simulink model "Target_Control_System"  (R2021b)
settings: Solver=FixedStepDiscrete  StartTime=0.0  StopTime=5  RelTol=1e-3
PreLoadFcn:
  | RTWConfigurationCB('preloadfcn', bdroot);
PostLoadFcn:
  | load('configuration/data_struct.mat');
  | load('configuration/fluxMaps_propMotor.mat');
  | load('configuration/parameterInit_PROP.mat');
  | load('configuration/parameterInit_PUMP.mat');
  | load('configuration/parameterInit_PITCH.mat');
  | load('configuration/parameterInit_TILT.mat');
  | %load('configuration/base_workspace_signal_definition.mat');
  | %load('resolvedatastores_to_baseworkspace_for_faster_simulation.mat');
model workspace (MAT data in the model file):
  SIMULATION_OPTIONS : Simulink.Parameter (value not decoded)
  TARGET_CODE_GEN : Simulink.Parameter (value not decoded)
  TCS_SAMPLE_FREQ_HZ : Simulink.Parameter (value not decoded)
symbols that are objects in the model workspace (value not decoded): TARGET_CODE_GEN, TCS_SAMPLE_FREQ_HZ
undefined symbols (not defined in the file): A_DQ_REF_LPF_INIT__PITCH, A_DQ_REF_LPF_INIT__PROP, A_DQ_REF_LPF_INIT__PUMP, A_DQ_REF_LPF_INIT__TILT, A_OBSERVER_CONFIDENCE_INIT__PITCH, A_OBSERVER_CONFIDENCE_INIT__PROP, A_OBSERVER_CONFIDENCE_INIT__PUMP, A_OBSERVER_CONFIDENCE_INIT__TILT, ACTUATOR_MAX_ANGLE_TRIP__PITCH, ACTUATOR_MIN_ANGLE_TRIP__PITCH, ACTUATOR_POS_SENSOR_INV_DIRECTION__PITCH, ACTUATOR_POS_SENSOR_INV_DIRECTION__TILT, ACTUATOR_POS_SENSOR_OFFSET__PITCH, ACTUATOR_POS_SENSOR_OFFSET__TILT, ADC_scaler1_baseaddr_TILT, ADC_SCALER_FLOAT_TO_FIXPOINT_EXPANSION, ANGLE_ELEC_FROM_SENSOR_OFFSET_INIT__PITCH, ANGLE_ELEC_FROM_SENSOR_OFFSET_INIT__PROP, ANGLE_ELEC_FROM_SENSOR_OFFSET_INIT__PUMP, ANGLE_ELEC_FROM_SENSOR_OFFSET_INIT__TILT, AUTO_CLEAR_FAULTS_ENABLED__PITCH, AUTO_CLEAR_FAULTS_ENABLED__PROP, AUTO_CLEAR_FAULTS_ENABLED__PUMP, AUTO_CLEAR_FAULTS_ENABLED__TILT, AUTO_CLEAR_FAULTS_WAIT_TICKS__PITCH, AUTO_CLEAR_FAULTS_WAIT_TICKS__PROP, AUTO_CLEAR_FAULTS_WAIT_TICKS__PUMP, AUTO_CLEAR_FAULTS_WAIT_TICKS__TILT, AUTO_I_ZERO_IDLE_TICKS__PITCH, AUTO_I_ZERO_IDLE_TICKS__PROP, AUTO_I_ZERO_IDLE_TICKS__PUMP, AUTO_I_ZERO_IDLE_TICKS__TILT, AUTO_I_ZERO_OFFSET_IDC_THRESHOLD__PITCH, AUTO_I_ZERO_OFFSET_IDC_THRESHOLD__PROP, AUTO_I_ZERO_OFFSET_IDC_THRESHOLD__PUMP, AUTO_I_ZERO_OFFSET_IDC_THRESHOLD__TILT, AUTO_I_ZERO_OFFSET_IPH_THRESHOLD__PITCH, AUTO_I_ZERO_OFFSET_IPH_THRESHOLD__PROP, AUTO_I_ZERO_OFFSET_IPH_THRESHOLD__PUMP, AUTO_I_ZERO_OFFSET_IPH_THRESHOLD__TILT, AUTO_SENSORLESS_SWITCHOVER_DISABLE_OMEGA, AUTO_SENSORLESS_SWITCHOVER_ENABLE_OMEGA, AUTO_SENSORLESS_SWITCHOVER_MIN_CONFIDENCE, AUXILIARY_PROTECTION_UNIT_BASEADDR__TILT, blanking_max_error_omega_INIT_PITCH, blanking_max_error_omega_INIT_TILT, blanking_max_error_position_INIT_PITCH, blanking_max_error_position_INIT_TILT, BRUTE_START_I_Q_REF_RAMP_SPEED__PITCH, BRUTE_START_I_Q_REF_RAMP_SPEED__PROP, BRUTE_START_I_Q_REF_RAMP_SPEED__PUMP, BRUTE_START_I_Q_REF_RAMP_SPEED__TILT, CONTROL_LOOP_DT_INIT__PITCH, CONTROL_LOOP_DT_INIT__PROP, CONTROL_LOOP_DT_INIT__PUMP, CONTROL_LOOP_DT_INIT__TILT, CORRECTION_FILTER_SCALE__PITCH, CORRECTION_FILTER_SCALE__PROP, CORRECTION_FILTER_SCALE__PUMP, CORRECTION_FILTER_SCALE__TILT ... (+458)
libraries: simulink x178, Reusables_Lib x24
(part 31 of 47)

== system Target_Control_System/Target_Control_System/Simulation Controls/Simulation Data Store Initialization/setPositionControlModeTilt()/Enabled Subsystem/Switch Case Action Subsystem ePassiveHolding ==
  Action Port : ActionPort
  Constant : Constant  Value=I_SET_MAX_PASSIVE_HOLDING__TILT  OutDataTypeStr=single
  Constant1 : Constant  Value=0  OutDataTypeStr=int32
  Constant2 : Constant  Value=0  OutDataTypeStr=uint32
  Constant3 : Constant  OutDataTypeStr=uint32
  Constant4 : Constant  OutDataTypeStr=uint32
  Data Store Write : DataStoreWrite  DataStoreName=oTilt  DataStoreElements=oTilt.oMot_.oParam_.fISetpointMax_  IndexOptions=Index vector (dialog)  Indices=1  OutputSizes=1
  Data Store Write1 : DataStoreWrite  DataStoreName=oTilt  DataStoreElements=oTilt.oMot_.oState_.oPosSensor_.iPosControlEnabled_  IndexOptions=Index vector (dialog)  Indices=1  OutputSizes=1
  Data Store Write2 : DataStoreWrite  DataStoreName=oTilt  DataStoreElements=oTilt.oMot_.oState_.uiSpeedControllerActive_  IndexOptions=Index vector (dialog)  Indices=1  OutputSizes=1
  Data Store Write3 : DataStoreWrite  DataStoreName=oTilt  DataStoreElements=oTilt.oMot_.oOut_.uiForcedAngle_  IndexOptions=Index vector (dialog)  Indices=1  OutputSizes=1
  Data Store Write4 : DataStoreWrite  DataStoreName=oTilt  DataStoreElements=oTilt.oMot_.oParam_.iForcedPositionHoldMode_  IndexOptions=Index vector (dialog)  Indices=1  OutputSizes=1
  wires:
  Constant/1 -> Data Store Write/1
  Constant1/1 -> Data Store Write1/1
  Constant2/1 -> Data Store Write2/1
  Constant3/1 -> Data Store Write3/1
  Constant4/1 -> Data Store Write4/1

== system Target_Control_System/Target_Control_System/Simulation Controls/Simulation Data Store Initialization/setPositionControlModeTilt()/Enabled Subsystem/Switch Case Action Subsystem eTorqueMirror ==
  note: // This is the only setting that directly matters for the torque mirror mode. // The remaining settings are set up because the position and speed control loops do run in the background for sanity checks
  Action Port : ActionPort
  Constant : Constant  Value=SLAVE_RPM_CTRL_INTEGRATOR_LEAKAGE_FACTOR__TILT  OutDataTypeStr=single
  Constant1 : Constant  Value=SLAVE_RPM_CTRL_ERROR_REDUCTION_RADS_PER_S__TILT  OutDataTypeStr=single
  Constant2 : Constant  Value=SLAVE_POS_CTRL_ERROR_REDUCTION_RAD__TILT  OutDataTypeStr=single
  Constant3 : Constant  OutDataTypeStr=uint32
  Data Store Write : DataStoreWrite  DataStoreName=oTilt  DataStoreElements=oTilt.oMot_.oParam_.oPid2DataRpmCtrl_.oParameter_.fIntegratorLeakFactor_  IndexOptions=Index vector (dialog)  Indices=1  OutputSizes=1
  Data Store Write1 : DataStoreWrite  DataStoreName=oTilt  DataStoreElements=oTilt.oMot_.oParam_.oPid2DataRpmCtrl_.oParameter_.fErrorReduction_  IndexOptions=Index vector (dialog)  Indices=1  OutputSizes=1
  Data Store Write2 : DataStoreWrite  DataStoreName=oTilt  DataStoreElements=oTilt.oMot_.oState_.oPosSensor_.oPidDataPosCtrl_.oParameter_.fErrorReduction_  IndexOptions=Index vector (dialog)  Indices=1  OutputSizes=1
  Data Store Write3 : DataStoreWrite  DataStoreName=oTilt  DataStoreElements=oTilt.oMot_.oParam_.uiTorqueMirroringActive_  IndexOptions=Index vector (dialog)  Indices=1  OutputSizes=1
  wires:
  Constant1/1 -> Data Store Write1/1
  Constant/1 -> Data Store Write/1
  Constant2/1 -> Data Store Write2/1
  Constant3/1 -> Data Store Write3/1

== system Target_Control_System/Target_Control_System/Simulation Controls/Simulation Data Store Initialization/setTiltMotorSpecificParameters()/Enabled Subsystem MotorType/Switch Case Action Subsystem MotorType12 ==
  note: // Current controller gains
  note: // Current maxima and dynamic limit
  note: // Speed controller gains
  note: // Maximum speeds
  note: // Position loop tweaks
  Action Port : ActionPort  ActionPortLabel=case [ 1 2 ]:
  Constant : Constant
  Constant1 : Constant  OutDataTypeStr=int32
  Constant10 : Constant  Value=IDC_MIN_TRIP_INIT__TILT_TIP  OutDataTypeStr=single
  Constant11 : Constant  Value=IDC_MAX_TRIP_INIT__TILT_TIP  OutDataTypeStr=single
  Constant12 : Constant  Commented=on  Value=I_MAX_WHILE_OFF_TILT_TIP  OutDataTypeStr=single
  Constant13 : Constant  Value=I_TRIP_HW_INIT__TILT_TIP  OutDataTypeStr=single
  Constant14 : Constant  Value=RPM_CTRL_KI_INIT__TILT_TIP  OutDataTypeStr=single
  Constant15 : Constant  Value=RPM_CTRL_KP_INIT__TILT_TIP  OutDataTypeStr=single
  Constant{16..17,19..20} (4 alike) : Constant  Value=RPM_CTRL_RAMP_SPEED_INIT_TILT_TIP  OutDataTypeStr=single
  Constant18 : Constant  Value=RPM_CTRL_KI_INIT__TILT_TIP  OutDataTypeStr=single
  Constant2 : Constant  Value=INPUT_TO_OUTPUT_SENSOR_MAX_DIFFERENCE_TRIP__TILT_TIP  OutDataTypeStr=single
  Constant21 : Constant  Value=POSITION_RAMP_UPSLOPE_RAD_PER_S_INIT__TILT_TIP  OutDataTypeStr=single
  Constant22 : Constant  Value=POSITION_RAMP_UPSLOPE_RAD_PER_S_INIT__TILT_TIP  OutDataTypeStr=single
  Constant23 : Constant  Value=0.10471975512  OutDataTypeStr=single
  Constant24 : Constant  Value=DUAL_SERVO_ALWAYS_MIRROR_ANG_ERR__TILT_TIP  OutDataTypeStr=single
  Constant25 : Constant  Value=DUAL_SERVO_IQ_SWITCHOVER_ERROR__TILT_TIP  OutDataTypeStr=single
  Constant26 : Constant  Value=DUAL_SERVO_CONDITIONALLY_MIRROR_ANG_ERR__TILT_TIP  OutDataTypeStr=single
  Constant3 : Constant  Value=I_CTRL_KP_INIT__TILT_TIP  OutDataTypeStr=single
  Constant4 : Constant  Value=I_CTRL_KI_INIT__TILT_TIP  OutDataTypeStr=single
  Constant5 : Constant  Value=DYNAMIC_I_LIM_I_MAX__TILT_TIP  OutDataTypeStr=single
  Constant6 : Constant  Value=DYNAMIC_I_LIM_BLEEDDOWN_FACTOR__TILT_TIP  OutDataTypeStr=single
  Constant7 : Constant  Value=DYNAMIC_I_LIM_KNOCKDOWN_FACTOR__TILT_TIP  OutDataTypeStr=single
  Constant8 : Constant  Value=I_SET_MAX_INIT__TILT_TIP  OutDataTypeStr=single
  Constant9 : Constant  Value=I_TRIP_SW_INIT__TILT_TIP  OutDataTypeStr=single
  Data Store Write : DataStoreWrite  DataStoreName=oTilt  DataStoreElements=oTilt.oMot_.oState_.oPosSensor_.iTiltReadheadCompensationEnabled_  IndexOptions=Index vector (dialog)  Indices=1  OutputSizes=1
  Data Store Write1 : DataStoreWrite  DataStoreName=oTilt  DataStoreElements=oTilt.oMot_.oState_.oPosSensor_.fInputToOutputSensorMaxDifference_  IndexOptions=Index vector (dialog)  Indices=1  OutputSizes=1
  Data Store Write10 : DataStoreWrite  DataStoreName=oTilt  DataStoreElements=oTilt.oMot_.oParam_.fTripLimitSoftwareA_  IndexOptions=Index vector (dialog)  Indices=1  OutputSizes=1
  Data Store Write11 : DataStoreWrite  DataStoreName=oTilt  DataStoreElements=oTilt.oMot_.oParam_.fIdcMinTrip_  IndexOptions=Index vector (dialog)  Indices=1  OutputSizes=1
  Data Store Write12 : DataStoreWrite  DataStoreName=oTilt  DataStoreElements=oTilt.oMot_.oParam_.fIdcMaxTrip_  IndexOptions=Index vector (dialog)  Indices=1  OutputSizes=1
  Data Store Write13 : DataStoreWrite  Commented=on  DataStoreName=oTilt  DataStoreElements=oTilt.oMot_.oParam_.fMaximumPhaseCurrentWhileOff_  IndexOptions=Index vector (dialog)  Indices=1  OutputSizes=1
  Data Store Write14 : DataStoreWrite  DataStoreName=oTilt  DataStoreElements=oTilt.oHw_.fTripLimitHardware_  IndexOptions=Index vector (dialog)  Indices=1  OutputSizes=1
  Data Store Write15 : DataStoreWrite  DataStoreName=oTilt  DataStoreElements=oTilt.oMot_.oParam_.oPid2DataRpmCtrl_.oParameter_.fKi_  IndexOptions=Index vector (dialog)  Indices=1  OutputSizes=1
  Data Store Write16 : DataStoreWrite  DataStoreName=oTilt  DataStoreElements=oTilt.oMot_.oParam_.oPid2DataRpmCtrl_.oParameter_.fKp_  IndexOptions=Index vector (dialog)  Indices=1  OutputSizes=1
  Data Store Write17 : DataStoreWrite  DataStoreName=oTilt  DataStoreElements=oTilt.oMot_.oState_.oRampDataOmegaERef_.oParam_.fUpslope_  IndexOptions=Index vector (dialog)  Indices=1  OutputSizes=1
  Data Store Write18 : DataStoreWrite  DataStoreName=oTilt  DataStoreElements=oTilt.oMot_.oState_.oRampDataOmegaERef_.oParam_.fDownslope_  IndexOptions=Index vector (dialog)  Indices=1  OutputSizes=1
  Data Store Write19 : DataStoreWrite  DataStoreName=oTilt  DataStoreElements=oTilt.oIsr_.oParam_.fOverspeedProtectionLimitOmegaE_  IndexOptions=Index vector (dialog)  Indices=1  OutputSizes=1
  Data Store Write2 : DataStoreWrite  DataStoreName=oTilt  DataStoreElements=oTilt.oIsr_.oParam_.oPiDataId_.oParameter_.fKp_  IndexOptions=Index vector (dialog)  Indices=1  OutputSizes=1
  Data Store Write20 : DataStoreWrite  DataStoreName=oTilt  DataStoreElements=oTilt.oMot_.oState_.oPosSensor_.oPidDataPosCtrl_.oParameter_.fOutMax_  IndexOptions=Index vector (dialog)  Indices=1  OutputSizes=1
  Data Store Write21 : DataStoreWrite  DataStoreName=oTilt  DataStoreElements=oTilt.oMot_.oState_.oPosSensor_.oPidDataPosCtrl_.oParameter_.fOutMin_  IndexOptions=Index vector (dialog)  Indices=1  OutputSizes=1
  Data Store Write22 : DataStoreWrite  DataStoreName=oTilt  DataStoreElements=oTilt.oMot_.oState_.oRampDataPos_.oParam_.fUpslope_  IndexOptions=Index vector (dialog)  Indices=1  OutputSizes=1
  Data Store Write23 : DataStoreWrite  DataStoreName=oTilt  DataStoreElements=oTilt.oMot_.oState_.oRampDataPos_.oParam_.fDownslope_  IndexOptions=Index vector (dialog)  Indices=1  OutputSizes=1
  Data Store Write24 : DataStoreWrite  DataStoreName=oTilt  DataStoreElements=oTilt.oMot_.oParam_.fDualServoAlwaysMirrorAngularError_  IndexOptions=Index vector (dialog)  Indices=1  OutputSizes=1
  Data Store Write25 : DataStoreWrite  DataStoreName=oTilt  DataStoreElements=oTilt.oMot_.oParam_.fDualServoIqSwitchoverError_  IndexOptions=Index vector (dialog)  Indices=1  OutputSizes=1
  Data Store Write26 : DataStoreWrite  DataStoreName=oTilt  DataStoreElements=oTilt.oMot_.oParam_.fDualServoConditionallyMirrorAngularError_  IndexOptions=Index vector (dialog)  Indices=1  OutputSizes=1
  Data Store Write3 : DataStoreWrite  DataStoreName=oTilt  DataStoreElements=oTilt.oIsr_.oParam_.oPiDataId_.oParameter_.fKi_  IndexOptions=Index vector (dialog)  Indices=1  OutputSizes=1
  Data Store Write4 : DataStoreWrite  DataStoreName=oTilt  DataStoreElements=oTilt.oIsr_.oParam_.oPiDataIq_.oParameter_.fKp_  IndexOptions=Index vector (dialog)  Indices=1  OutputSizes=1
  Data Store Write5 : DataStoreWrite  DataStoreName=oTilt  DataStoreElements=oTilt.oIsr_.oParam_.oPiDataIq_.oParameter_.fKi_  IndexOptions=Index vector (dialog)  Indices=1  OutputSizes=1
  Data Store Write6 : DataStoreWrite  DataStoreName=oTilt  DataStoreElements=oTilt.oMot_.oParam_.fDynILimDynamicMax_  IndexOptions=Index vector (dialog)  Indices=1  OutputSizes=1
  Data Store Write7 : DataStoreWrite  DataStoreName=oTilt  DataStoreElements=oTilt.oMot_.oParam_.fDynILimIntegratorLeakageFactor_  IndexOptions=Index vector (dialog)  Indices=1  OutputSizes=1
  Data Store Write8 : DataStoreWrite  DataStoreName=oTilt  DataStoreElements=oTilt.oMot_.oParam_.fDynILimKnockdownFactor_  IndexOptions=Index vector (dialog)  Indices=1  OutputSizes=1
  Data Store Write9 : DataStoreWrite  Commented=on  DataStoreName=oTilt  DataStoreElements=oTilt.oMot_.oParam_.fISetpointMax_  IndexOptions=Index vector (dialog)  Indices=1  OutputSizes=1
  Merge : Merge
  Merge1 : Merge
  Multiply : Product  Inputs=**
  Switch Case : SwitchCase  CaseConditions={1,2}  ShowDefaultCase=off
  Switch Case Action Subsystem Motor Type1 : Subsystem  TreatAsAtomicUnit=on
  Switch Case Action Subsystem Motor Type2 : Subsystem  TreatAsAtomicUnit=on
  Unary Minus : UnaryMinus
  IsetpointMax : Outport
  maxTrip : Outport  Port=2
  minTrip : Outport  Port=3
  wires:
  Unary Minus/1 -> Data Store Write21/1
  Constant22/1 -> Data Store Write23/1
  Constant11/1 -> Data Store Write12/1
  Constant18/1 -> Multiply/1
  Constant21/1 -> Data Store Write22/1
  Constant3/1 -> Data Store Write4/1, Data Store Write2/1
  Constant7/1 -> Data Store Write8/1
  Constant12/1 -> Data Store Write13/1
  Constant10/1 -> Data Store Write11/1
  Multiply/1 -> Data Store Write19/1
  Constant16/1 -> Data Store Write17/1
  Constant26/1 -> Data Store Write26/1
  Constant9/1 -> Data Store Write10/1
  Constant4/1 -> Data Store Write5/1, Data Store Write3/1
  Constant6/1 -> Data Store Write7/1
  Constant20/1 -> Unary Minus/1
  Constant25/1 -> Data Store Write25/1
  Constant17/1 -> Data Store Write18/1
  Constant19/1 -> Data Store Write20/1
  Constant13/1 -> Data Store Write14/1
  Constant8/1 -> IsetpointMax/1, Data Store Write9/1
  Constant5/1 -> Data Store Write6/1
  Constant24/1 -> Data Store Write24/1
  Constant2/1 -> Data Store Write1/1
  Constant23/1 -> Multiply/2
  Constant14/1 -> Data Store Write15/1
  Constant15/1 -> Data Store Write16/1
  Constant1/1 -> Data Store Write/1
  Constant/1 -> Switch Case/1
  Switch Case/1 -> Switch Case Action Subsystem Motor Type1/Action
  Switch Case/2 -> Switch Case Action Subsystem Motor Type2/Action
  Switch Case Action Subsystem Motor Type1/1(maxTrip) -> Merge/2
  Switch Case Action Subsystem Motor Type2/1(maxTrip) -> Merge/1
  Merge/1 -> maxTrip/1
  Switch Case Action Subsystem Motor Type1/2(minTrip) -> Merge1/1
  Switch Case Action Subsystem Motor Type2/2(minTrip) -> Merge1/2
  Merge1/1 -> minTrip/1

== system Target_Control_System/Target_Control_System/Simulation Controls/Simulation Data Store Initialization/setTiltMotorSpecificParameters()/Enabled Subsystem MotorType/Switch Case Action Subsystem MotorType3 ==
  note: // This is a linkage style tilt, both sensors directly read the harmonic drive output angle (after the calculated gearbox) // but before the linkage. They will move over about 200°. 0 is defined to be cruise.
  note: // Maximum speeds
  note: // Speed controller gains
  note: // Current maxima and dynamic limit
  note: // Current controller gains
  note: // Position loop tweaks
  Action Port : ActionPort  ActionPortLabel=case [ 3 ]:
  Constant : Constant  Value=IQ_REF_FILTER_FOR_SPEED_CONTROL_BW_3DB_HZ__TILT_LINAKGE  OutDataTypeStr=single
  Constant1 : Constant  Value=0  OutDataTypeStr=int32
  Constant10 : Constant  Value=IDC_MIN_TRIP_INIT__TILT_LINKAGE  OutDataTypeStr=single
  Constant11 : Constant  Value=IDC_MAX_TRIP_INIT__TILT_LINKAGE  OutDataTypeStr=single
  Constant12 : Constant  Commented=on  Value=I_MAX_WHILE_OFF_TILT_LINKAGE  OutDataTypeStr=single
  Constant13 : Constant  Value=I_TRIP_HW_INIT__TILT_LINKAGE  OutDataTypeStr=single
  Constant14 : Constant  Value=RPM_CTRL_KI_INIT__TILT_LINKAGE  OutDataTypeStr=single
  Constant15 : Constant  Value=RPM_CTRL_KP_INIT__TILT_LINKAGE  OutDataTypeStr=single
  Constant{16..17,19..20} (4 alike) : Constant  Value=RPM_CTRL_RAMP_SPEED_INIT_TILT_LINKAGE  OutDataTypeStr=single
  Constant18 : Constant  Value=RPM_CTRL_KI_INIT__TILT_LINKAGE  OutDataTypeStr=single
  Constant2 : Constant  Value=INPUT_TO_OUTPUT_SENSOR_MAX_DIFFERENCE_TRIP__TILT_LINKAGE  OutDataTypeStr=single
  Constant21 : Constant  Value=POSITION_RAMP_UPSLOPE_RAD_PER_S_INIT__TILT_LINKAGE  OutDataTypeStr=single
  Constant22 : Constant  Value=POSITION_RAMP_UPSLOPE_RAD_PER_S_INIT__TILT_LINKAGE  OutDataTypeStr=single
  Constant23 : Constant  Value=0.10471975512  OutDataTypeStr=single
  Constant24 : Constant  Value=DUAL_SERVO_ALWAYS_MIRROR_ANG_ERR__TILT_LINKAGE  OutDataTypeStr=single
  Constant25 : Constant  Value=DUAL_SERVO_IQ_SWITCHOVER_ERROR__TILT_LINKAGE  OutDataTypeStr=single
  Constant26 : Constant  Value=DUAL_SERVO_CONDITIONALLY_MIRROR_ANG_ERR__TILT_LINKAGE  OutDataTypeStr=single
  Constant27 : Constant  Value=POSITION_CONTROL_SETMIN__TILT_LINKAGE  OutDataTypeStr=single
  Constant28 : Constant  Value=POSITION_CONTROL_SETMAX__TILT_LINKAGE  OutDataTypeStr=single
  Constant29 : Constant  Value=GBX_MAX_ANGLE_TRIP__TILT_LINKAGE  OutDataTypeStr=single
  Constant3 : Constant  Value=I_CTRL_KP_INIT__TILT_LINKAGE  OutDataTypeStr=single
  Constant30 : Constant  Value=GBX_MIN_ANGLE_TRIP__TILT_LINKAGE  OutDataTypeStr=single
  Constant31 : Constant  Value=161.0  OutDataTypeStr=single
  Constant32 : Constant  Value=POS_KP_INIT__TILT_LINKAGE  OutDataTypeStr=single
  Constant33 : Constant  OutDataTypeStr=single
  Constant4 : Constant  Value=I_CTRL_KI_INIT__TILT_LINKAGE  OutDataTypeStr=single
  Constant5 : Constant  Value=DYNAMIC_I_LIM_I_MAX__TILT_LINKAGE  OutDataTypeStr=single
  Constant6 : Constant  Value=DYNAMIC_I_LIM_BLEEDDOWN_FACTOR__TILT_LINKAGE  OutDataTypeStr=single
  Constant7 : Constant  Value=DYNAMIC_I_LIM_KNOCKDOWN_FACTOR__TILT_LINKAGE  OutDataTypeStr=single
  Constant8 : Constant  Value=I_SET_MAX_INIT__TILT_LINKAGE  OutDataTypeStr=single
  Constant9 : Constant  Value=I_TRIP_SW_INIT__TILT_LINKAGE  OutDataTypeStr=single
  Data Store Read : DataStoreRead  DataStoreName=oTilt  DataStoreElements=oTilt.oIsr_.oParam_.fControlLoopDt_  IndexOptions=Index vector (dialog)  Indices=1  OutputSizes=1
  Data Store Write : DataStoreWrite  DataStoreName=oTilt  DataStoreElements=oTilt.oMot_.oState_.oPosSensor_.iTiltReadheadCompensationEnabled_  IndexOptions=Index vector (dialog)  Indices=1  OutputSizes=1
  Data Store Write1 : DataStoreWrite  DataStoreName=oTilt  DataStoreElements=oTilt.oMot_.oState_.oPosSensor_.fInputToOutputSensorMaxDifference_  IndexOptions=Index vector (dialog)  Indices=1  OutputSizes=1
  Data Store Write10 : DataStoreWrite  DataStoreName=oTilt  DataStoreElements=oTilt.oMot_.oParam_.fTripLimitSoftwareA_  IndexOptions=Index vector (dialog)  Indices=1  OutputSizes=1
  Data Store Write11 : DataStoreWrite  DataStoreName=oTilt  DataStoreElements=oTilt.oMot_.oParam_.fIdcMinTrip_  IndexOptions=Index vector (dialog)  Indices=1  OutputSizes=1
  Data Store Write12 : DataStoreWrite  DataStoreName=oTilt  DataStoreElements=oTilt.oMot_.oParam_.fIdcMaxTrip_  IndexOptions=Index vector (dialog)  Indices=1  OutputSizes=1
  Data Store Write13 : DataStoreWrite  Commented=on  DataStoreName=oTilt  DataStoreElements=oTilt.oMot_.oParam_.fMaximumPhaseCurrentWhileOff_  IndexOptions=Index vector (dialog)  Indices=1  OutputSizes=1
  Data Store Write14 : DataStoreWrite  DataStoreName=oTilt  DataStoreElements=oTilt.oHw_.fTripLimitHardware_  IndexOptions=Index vector (dialog)  Indices=1  OutputSizes=1
  Data Store Write15 : DataStoreWrite  DataStoreName=oTilt  DataStoreElements=oTilt.oMot_.oParam_.oPid2DataRpmCtrl_.oParameter_.fKi_  IndexOptions=Index vector (dialog)  Indices=1  OutputSizes=1
  Data Store Write16 : DataStoreWrite  DataStoreName=oTilt  DataStoreElements=oTilt.oMot_.oParam_.oPid2DataRpmCtrl_.oParameter_.fKp_  IndexOptions=Index vector (dialog)  Indices=1  OutputSizes=1
  Data Store Write17 : DataStoreWrite  DataStoreName=oTilt  DataStoreElements=oTilt.oMot_.oState_.oRampDataOmegaERef_.oParam_.fUpslope_  IndexOptions=Index vector (dialog)  Indices=1  OutputSizes=1
  Data Store Write18 : DataStoreWrite  DataStoreName=oTilt  DataStoreElements=oTilt.oMot_.oState_.oRampDataOmegaERef_.oParam_.fDownslope_  IndexOptions=Index vector (dialog)  Indices=1  OutputSizes=1
  Data Store Write19 : DataStoreWrite  DataStoreName=oTilt  DataStoreElements=oTilt.oIsr_.oParam_.fOverspeedProtectionLimitOmegaE_  IndexOptions=Index vector (dialog)  Indices=1  OutputSizes=1
  Data Store Write2 : DataStoreWrite  DataStoreName=oTilt  DataStoreElements=oTilt.oIsr_.oParam_.oPiDataId_.oParameter_.fKp_  IndexOptions=Index vector (dialog)  Indices=1  OutputSizes=1
  Data Store Write20 : DataStoreWrite  DataStoreName=oTilt  DataStoreElements=oTilt.oMot_.oState_.oPosSensor_.oPidDataPosCtrl_.oParameter_.fOutMax_  IndexOptions=Index vector (dialog)  Indices=1  OutputSizes=1
  Data Store Write21 : DataStoreWrite  DataStoreName=oTilt  DataStoreElements=oTilt.oMot_.oState_.oPosSensor_.oPidDataPosCtrl_.oParameter_.fOutMin_  IndexOptions=Index vector (dialog)  Indices=1  OutputSizes=1
  Data Store Write22 : DataStoreWrite  DataStoreName=oTilt  DataStoreElements=oTilt.oMot_.oState_.oRampDataPos_.oParam_.fUpslope_  IndexOptions=Index vector (dialog)  Indices=1  OutputSizes=1
  Data Store Write23 : DataStoreWrite  DataStoreName=oTilt  DataStoreElements=oTilt.oMot_.oState_.oRampDataPos_.oParam_.fDownslope_  IndexOptions=Index vector (dialog)  Indices=1  OutputSizes=1
  Data Store Write24 : DataStoreWrite  DataStoreName=oTilt  DataStoreElements=oTilt.oMot_.oParam_.fDualServoAlwaysMirrorAngularError_  IndexOptions=Index vector (dialog)  Indices=1  OutputSizes=1
  Data Store Write25 : DataStoreWrite  DataStoreName=oTilt  DataStoreElements=oTilt.oMot_.oParam_.fDualServoIqSwitchoverError_  IndexOptions=Index vector (dialog)  Indices=1  OutputSizes=1
  Data Store Write26 : DataStoreWrite  DataStoreName=oTilt  DataStoreElements=oTilt.oMot_.oParam_.fDualServoConditionallyMirrorAngularError_  IndexOptions=Index vector (dialog)  Indices=1  OutputSizes=1
  Data Store Write27 : DataStoreWrite  DataStoreName=oTilt  DataStoreElements=oTilt.oMot_.oParam_.fPositionSetpointMin_  IndexOptions=Index vector (dialog)  Indices=1  OutputSizes=1
  Data Store Write28 : DataStoreWrite  DataStoreName=oTilt  DataStoreElements=oTilt.oMot_.oParam_.fPositionSetpointMax_  IndexOptions=Index vector (dialog)  Indices=1  OutputSizes=1
  Data Store Write29 : DataStoreWrite  Commented=on  DataStoreName=oTilt  DataStoreElements=oTilt.oMot_.oState_.oPosSensor_.fGbxAngleMaxTrip_  IndexOptions=Index vector (dialog)  Indices=1  OutputSizes=1
  Data Store Write3 : DataStoreWrite  DataStoreName=oTilt  DataStoreElements=oTilt.oIsr_.oParam_.oPiDataId_.oParameter_.fKi_  IndexOptions=Index vector (dialog)  Indices=1  OutputSizes=1
  Data Store Write30 : DataStoreWrite  Commented=on  DataStoreName=oTilt  DataStoreElements=oTilt.oMot_.oState_.oPosSensor_.fGbxAngleMinTrip_  IndexOptions=Index vector (dialog)  Indices=1  OutputSizes=1
  Data Store Write31 : DataStoreWrite  DataStoreName=oTilt  DataStoreElements=oTilt.oMot_.oState_.oPosSensor_.oGbx_.fGbxRatio_  IndexOptions=Index vector (dialog)  Indices=1  OutputSizes=1
  Data Store Write32 : DataStoreWrite  DataStoreName=oTilt  DataStoreElements=oTilt.oMot_.oState_.oPosSensor_.oPidDataPosCtrl_.oParameter_.fKp_  IndexOptions=Index vector (dialog)  Indices=1  OutputSizes=1
  Data Store Write33 : DataStoreWrite  DataStoreName=oTilt  DataStoreElements=oTilt.oMot_.oState_.fFilterBandwidthForSpeedControlIqRef_  IndexOptions=Index vector (dialog)  Indices=1  OutputSizes=1
  Data Store Write4 : DataStoreWrite  DataStoreName=oTilt  DataStoreElements=oTilt.oIsr_.oParam_.oPiDataIq_.oParameter_.fKp_  IndexOptions=Index vector (dialog)  Indices=1  OutputSizes=1
  Data Store Write5 : DataStoreWrite  DataStoreName=oTilt  DataStoreElements=oTilt.oIsr_.oParam_.oPiDataIq_.oParameter_.fKi_  IndexOptions=Index vector (dialog)  Indices=1  OutputSizes=1
  Data Store Write6 : DataStoreWrite  DataStoreName=oTilt  DataStoreElements=oTilt.oMot_.oParam_.fDynILimDynamicMax_  IndexOptions=Index vector (dialog)  Indices=1  OutputSizes=1
  Data Store Write7 : DataStoreWrite  DataStoreName=oTilt  DataStoreElements=oTilt.oMot_.oParam_.fDynILimIntegratorLeakageFactor_  IndexOptions=Index vector (dialog)  Indices=1  OutputSizes=1
  Data Store Write8 : DataStoreWrite  DataStoreName=oTilt  DataStoreElements=oTilt.oMot_.oParam_.fDynILimKnockdownFactor_  IndexOptions=Index vector (dialog)  Indices=1  OutputSizes=1
  Data Store Write9 : DataStoreWrite  Commented=on  DataStoreName=oTilt  DataStoreElements=oTilt.oMot_.oParam_.fISetpointMax_  IndexOptions=Index vector (dialog)  Indices=1  OutputSizes=1
  Divide : Product  Inputs=*/
  Multiply : Product  Inputs=**
  softwareIirFilterInitialize() : Subsystem  Priority=15  TreatAsAtomicUnit=on
  IsetpointMax : Outport
  maxTrip : Outport  Port=2
  minTrip : Outport  Port=3
  wires:
  Constant8/1 -> IsetpointMax/1, Data Store Write9/1
  Constant14/1 -> Data Store Write15/1
  Constant24/1 -> Data Store Write24/1
  Constant25/1 -> Data Store Write25/1
  Constant23/1 -> Multiply/2
  Constant20/1 -> Data Store Write21/1
  Constant19/1 -> Data Store Write20/1
  Constant9/1 -> Data Store Write10/1
  Constant4/1 -> Data Store Write5/1, Data Store Write3/1
  Constant13/1 -> Data Store Write14/1
  Constant11/1 -> Data Store Write12/1
  Constant2/1 -> Data Store Write1/1
  Constant5/1 -> Data Store Write6/1
  Constant10/1 -> Data Store Write11/1
  Constant7/1 -> Data Store Write8/1
  Constant18/1 -> Multiply/1
  Multiply/1 -> Data Store Write19/1
  Constant3/1 -> Data Store Write4/1, Data Store Write2/1
  Constant22/1 -> Data Store Write23/1
  Constant6/1 -> Data Store Write7/1
  Constant12/1 -> Data Store Write13/1
  Constant16/1 -> Data Store Write17/1
  Constant21/1 -> Data Store Write22/1
  Constant17/1 -> Data Store Write18/1
  Constant15/1 -> Data Store Write16/1
  Constant26/1 -> Data Store Write26/1
  Constant1/1 -> Data Store Write/1
  Constant30/1 -> minTrip/1, Data Store Write30/1
  Constant29/1 -> maxTrip/1, Data Store Write29/1
  Constant28/1 -> Data Store Write28/1
  Constant27/1 -> Data Store Write27/1
  Constant31/1 -> Data Store Write31/1
  Constant32/1 -> Data Store Write32/1
  softwareIirFilterInitialize()/1(fActualFrequencyHz) -> Data Store Write33/1
  Constant/1 -> softwareIirFilterInitialize()/1(fFreq3db)
  Divide/1 -> softwareIirFilterInitialize()/2(fFreqSample)
  Data Store Read/1 -> Divide/2
  Constant33/1 -> Divide/1

== system Target_Control_System/Target_Control_System/Simulation Controls/Simulation Data Store Initialization/setupIirFilters(&oTilt)/softwareIirFilterInitialize()/computeCoefficientsButter() ==
  fCutoffFrequencyHz : Inport  OutDataTypeStr=single
  dSampleFrequencyHz : Inport  Port=2  OutDataTypeStr=single
  Add : Sum  Inputs=+++  OutDataTypeStr=double
  Add1 : Sum  Inputs=-+
  Add2 : Sum  Inputs=+-+  OutDataTypeStr=double
  Constant : Constant  Value=0.0008  OutDataTypeStr=single  SampleTime=-1
  Constant1 : Constant  Value=0.45  OutDataTypeStr=single  SampleTime=-1
  Constant{5,7,9..10} (4 alike) : Constant  SampleTime=-1
  Constant2 : Constant  Value=pi  OutDataTypeStr=double  SampleTime=-1
  Constant3 : Constant  OutDataTypeStr=double  SampleTime=-1
  Constant4 : Constant  Value=sqrt(2)  OutDataTypeStr=double  SampleTime=-1
  Constant6 : Constant  OutDataTypeStr=double  SampleTime=-1
  Constant8 : Constant  Value=2  SampleTime=-1
  Data Type Conversion : DataTypeConversion  OutDataTypeStr=double
  Divide : Product  Inputs=**  OutDataTypeStr=single
  Divide1 : Product  Inputs=**  OutDataTypeStr=single
  Divide{3,5..6,8,10..11} (6 alike) : Product  Inputs=**  OutDataTypeStr=double
  Divide2 : Product  Inputs=*/  OutDataTypeStr=double
  Divide4 : Product  Inputs=*/  OutDataTypeStr=double
  Divide7 : Product  Inputs=*/  OutDataTypeStr=double
  Divide9 : Product  Inputs=***  OutDataTypeStr=double
  Gain : Gain  Gain=2  OutDataTypeStr=double
  Gain1 : Gain  Gain=-1  OutDataTypeStr=double
  Gain2 : Gain  Gain=-1  OutDataTypeStr=double
  Gain3 : Gain  Gain=-1  OutDataTypeStr=double
  Mux : Mux  Inputs=6
  Saturation Dynamic : simulink/Discontinuities/Saturation Dynamic  OutMin=[]  OutMax=[]  OutDataTypeStr=Inherit: Same as second input  OutDataType=fixdt(1, 16)  OutScaling=2^-10  DoSatur=off
  Tan : Trigonometry  Operator=tan
  dpOutArray : Outport
  fFreq3db : Outport  Port=2
  wires:
  Saturation Dynamic/1 -> Data Type Conversion/1, fFreq3db/1  "fCutoffFrequencyHz"
  Data Type Conversion/1 -> Divide2/1
  Constant10/1 -> Mux/4
  [dA2] -> Gain3/1
  Gain3/1 -> Mux/6
  [dA1] -> Gain2/1
  Gain2/1 -> Mux/5
  [dB2] -> Mux/3
  [dB1] -> Mux/2
  [dB0] -> Mux/1
  Divide11/1 -> [dA2]
  Gain1/1 -> Divide11/2
  Add2/1 -> Gain1/1
  Constant9/1 -> Add2/3
  Divide10/1 -> Add2/2
  [kdQ] -> Divide10/2
  Constant7/1 -> Add1/1
  Divide8/1 -> Add1/2, Add2/1
  Divide9/1 -> [dA1]
  Constant8/1 -> Divide9/3
  Add1/1 -> Divide9/2
  [kdIta] -> Divide8/1, Divide8/2, Divide10/1
  Gain/1 -> [dB1]
  Divide7/1 -> [dB0], Gain/1, [dB2], Divide9/1, Divide11/1
  Add/1 -> Divide7/2
  Constant6/1 -> Divide7/1
  Constant5/1 -> Add/3
  Divide5/1 -> Add/2
  Divide6/1 -> Add/1
  [kdQ] -> Divide5/2
  [kdIta] -> Divide5/1, Divide6/1, Divide6/2
  Mux/1 -> dpOutArray/1
  Constant4/1 -> [kdQ]
  Divide4/1 -> [kdIta]
  Constant3/1 -> Divide4/1
  Tan/1 -> Divide4/2
  Divide3/1 -> Tan/1
  Constant2/1 -> Divide3/2
  Divide2/1 -> Divide3/1  "dFf"
  Constant/1 -> Divide/2
  fCutoffFrequencyHz/1 -> Saturation Dynamic/2  "fCutoffFrequencyHz"
  Divide1/1 -> Saturation Dynamic/1
  dSampleFrequencyHz/1 -> Divide1/2, Divide2/2, Divide/1
  Constant1/1 -> Divide1/1
  Divide/1 -> Saturation Dynamic/3

== system Target_Control_System/Target_Control_System/Simulation Controls/Simulation Data Store Initialization/setupIirFilters()/softwareIirFilterInitialize()/computeCoefficientsButter() ==
  fCutoffFrequencyHz : Inport  OutDataTypeStr=single
  dSampleFrequencyHz : Inport  Port=2  OutDataTypeStr=single
  Add : Sum  Inputs=+++  OutDataTypeStr=double
  Add1 : Sum  Inputs=-+
  Add2 : Sum  Inputs=+-+  OutDataTypeStr=double
  Constant : Constant  Value=0.0008  OutDataTypeStr=single  SampleTime=-1
  Constant1 : Constant  Value=0.45  OutDataTypeStr=single  SampleTime=-1
  Constant{5,7,9..10} (4 alike) : Constant  SampleTime=-1
  Constant2 : Constant  Value=pi  OutDataTypeStr=double  SampleTime=-1
  Constant3 : Constant  OutDataTypeStr=double  SampleTime=-1
  Constant4 : Constant  Value=sqrt(2)  OutDataTypeStr=double  SampleTime=-1
  Constant6 : Constant  OutDataTypeStr=double  SampleTime=-1
  Constant8 : Constant  Value=2  SampleTime=-1
  Data Type Conversion : DataTypeConversion  OutDataTypeStr=double
  Divide : Product  Inputs=**  OutDataTypeStr=single
  Divide1 : Product  Inputs=**  OutDataTypeStr=single
  Divide{3,5..6,8,10..11} (6 alike) : Product  Inputs=**  OutDataTypeStr=double
  Divide2 : Product  Inputs=*/  OutDataTypeStr=double
  Divide4 : Product  Inputs=*/  OutDataTypeStr=double
  Divide7 : Product  Inputs=*/  OutDataTypeStr=double
  Divide9 : Product  Inputs=***  OutDataTypeStr=double
  Gain : Gain  Gain=2  OutDataTypeStr=double
  Gain1 : Gain  Gain=-1  OutDataTypeStr=double
  Gain2 : Gain  Gain=-1  OutDataTypeStr=double
  Gain3 : Gain  Gain=-1  OutDataTypeStr=double
  Mux : Mux  Inputs=6
  Saturation Dynamic : simulink/Discontinuities/Saturation Dynamic  OutMin=[]  OutMax=[]  OutDataTypeStr=Inherit: Same as second input  OutDataType=fixdt(1, 16)  OutScaling=2^-10  DoSatur=off
  Tan : Trigonometry  Operator=tan
  dpOutArray : Outport
  fFreq3db : Outport  Port=2
  wires:
  Saturation Dynamic/1 -> Data Type Conversion/1, fFreq3db/1  "fCutoffFrequencyHz"
  Data Type Conversion/1 -> Divide2/1
  Constant10/1 -> Mux/4
  [dA2] -> Gain3/1
  Gain3/1 -> Mux/6
  [dA1] -> Gain2/1
  Gain2/1 -> Mux/5
  [dB2] -> Mux/3
  [dB1] -> Mux/2
  [dB0] -> Mux/1
  Divide11/1 -> [dA2]
  Gain1/1 -> Divide11/2
  Add2/1 -> Gain1/1
  Constant9/1 -> Add2/3
  Divide10/1 -> Add2/2
  [kdQ] -> Divide10/2
  Constant7/1 -> Add1/1
  Divide8/1 -> Add1/2, Add2/1
  Divide9/1 -> [dA1]
  Constant8/1 -> Divide9/3
  Add1/1 -> Divide9/2
  [kdIta] -> Divide8/1, Divide8/2, Divide10/1
  Gain/1 -> [dB1]
  Divide7/1 -> [dB0], Gain/1, [dB2], Divide9/1, Divide11/1
  Add/1 -> Divide7/2
  Constant6/1 -> Divide7/1
  Constant5/1 -> Add/3
  Divide5/1 -> Add/2
  Divide6/1 -> Add/1
  [kdQ] -> Divide5/2
  [kdIta] -> Divide5/1, Divide6/1, Divide6/2
  Mux/1 -> dpOutArray/1
  Constant4/1 -> [kdQ]
  Divide4/1 -> [kdIta]
  Constant3/1 -> Divide4/1
  Tan/1 -> Divide4/2
  Divide3/1 -> Tan/1
  Constant2/1 -> Divide3/2
  Divide2/1 -> Divide3/1  "dFf"
  Constant/1 -> Divide/2
  fCutoffFrequencyHz/1 -> Saturation Dynamic/2  "fCutoffFrequencyHz"
  Divide1/1 -> Saturation Dynamic/1
  dSampleFrequencyHz/1 -> Divide1/2, Divide2/2, Divide/1
  Constant1/1 -> Divide1/1
  Divide/1 -> Saturation Dynamic/3

== system Target_Control_System/Target_Control_System/Simulation Controls/Simulation Data Store Initialization/setupObserverForPosSensor(&oTilt)/softwareIirFilterInitialize()/computeCoefficientsButter() ==
  fCutoffFrequencyHz : Inport  OutDataTypeStr=single
  dSampleFrequencyHz : Inport  Port=2  OutDataTypeStr=single
  Add : Sum  Inputs=+++  OutDataTypeStr=double
  Add1 : Sum  Inputs=-+
  Add2 : Sum  Inputs=+-+  OutDataTypeStr=double
  Constant : Constant  Value=0.0008  OutDataTypeStr=single
  Constant1 : Constant  Value=0.45  OutDataTypeStr=single
  Constant{5,7,9..10} (4 alike) : Constant
  Constant2 : Constant  Value=pi  OutDataTypeStr=double
  Constant3 : Constant  OutDataTypeStr=double
  Constant4 : Constant  Value=sqrt(2)  OutDataTypeStr=double
  Constant6 : Constant  OutDataTypeStr=double
  Constant8 : Constant  Value=2
  Data Type Conversion : DataTypeConversion  OutDataTypeStr=double
  Divide : Product  Inputs=**  OutDataTypeStr=single
  Divide1 : Product  Inputs=**  OutDataTypeStr=single
  Divide{3,5..6,8,10..11} (6 alike) : Product  Inputs=**  OutDataTypeStr=double
  Divide2 : Product  Inputs=*/  OutDataTypeStr=double
  Divide4 : Product  Inputs=*/  OutDataTypeStr=double
  Divide7 : Product  Inputs=*/  OutDataTypeStr=double
  Divide9 : Product  Inputs=***  OutDataTypeStr=double
  Gain : Gain  Gain=2  OutDataTypeStr=double
  Gain1 : Gain  Gain=-1  OutDataTypeStr=double
  Gain2 : Gain  Gain=-1  OutDataTypeStr=double
  Gain3 : Gain  Gain=-1  OutDataTypeStr=double
  Mux : Mux  Inputs=6
  Saturation Dynamic : simulink/Discontinuities/Saturation Dynamic  OutMin=[]  OutMax=[]  OutDataTypeStr=Inherit: Same as second input  OutDataType=fixdt(1, 16)  OutScaling=2^-10  DoSatur=off
  Tan : Trigonometry  Operator=tan
  dpOutArray : Outport
  fFreq3db : Outport  Port=2
  wires:
  Data Type Conversion/1 -> Divide2/1
  Constant10/1 -> Mux/4
  [dA2] -> Gain3/1
  Gain3/1 -> Mux/6
  [dA1] -> Gain2/1
  Gain2/1 -> Mux/5
  [dB2] -> Mux/3
  [dB1] -> Mux/2
  [dB0] -> Mux/1
  Divide11/1 -> [dA2]
  Gain1/1 -> Divide11/2
  Add2/1 -> Gain1/1
  Constant9/1 -> Add2/3
  Divide10/1 -> Add2/2
  [kdQ] -> Divide10/2
  Constant7/1 -> Add1/1
  Divide8/1 -> Add1/2, Add2/1
  Divide9/1 -> [dA1]
  Constant8/1 -> Divide9/3
  Add1/1 -> Divide9/2
  [kdIta] -> Divide8/1, Divide8/2, Divide10/1
  Gain/1 -> [dB1]
  Divide7/1 -> [dB0], Gain/1, [dB2], Divide9/1, Divide11/1
  Add/1 -> Divide7/2
  Constant6/1 -> Divide7/1
  Constant5/1 -> Add/3
  Divide5/1 -> Add/2
  Divide6/1 -> Add/1
  [kdQ] -> Divide5/2
  [kdIta] -> Divide5/1, Divide6/1, Divide6/2
  Mux/1 -> dpOutArray/1
  Constant4/1 -> [kdQ]
  Divide4/1 -> [kdIta]
  Constant3/1 -> Divide4/1
  Tan/1 -> Divide4/2
  Divide3/1 -> Tan/1
  Constant2/1 -> Divide3/2
  Divide2/1 -> Divide3/1  "dFf"
  Constant/1 -> Divide/2
  Saturation Dynamic/1 -> fFreq3db/1, Data Type Conversion/1  "fCutoffFrequencyHz"
  Divide1/1 -> Saturation Dynamic/1
  dSampleFrequencyHz/1 -> Divide1/2, Divide2/2, Divide/1
  Constant1/1 -> Divide1/1
  Divide/1 -> Saturation Dynamic/3
  fCutoffFrequencyHz/1 -> Saturation Dynamic/2

== system Target_Control_System/Target_Control_System/Simulation Controls/Simulation Data Store Initialization/setupPwm(&oTilt)/setPwmFrequencyApplication()_tilt/setPwmFrequency()_tilt ==
  fPwmFreqKhz_ : Inport
  fMotorAccelerationStage1Bandwidth_ : Inport  Port=2
  fFilterBandwidthForSpeedControlIqRef_ : Inport  Port=3
  Constant : Constant  Priority=1  Value=50000  OutDataTypeStr=single
  Constant1 : Constant  Priority=1  Value=0.0005  OutDataTypeStr=single
  Constant2 : Constant  Priority=1  OutDataTypeStr=single
  Data Store Read1 : DataStoreRead  Priority=1  DataStoreName=oTilt  DataStoreElements=oTilt.oMot_.oParam_.fObserverLoopFilterBandwidthHz_  IndexOptions=Index vector (dialog)  Indices=1  OutputSizes=1
  Data Store Read2 : DataStoreRead  Priority=1  DataStoreName=oTilt  DataStoreElements=oTilt.oMot_.oState_.oPosSensor_.fOmegaEDifferentiatorBandwidthHz_  IndexOptions=Index vector (dialog)  Indices=1  OutputSizes=1
  Data Store Write : DataStoreWrite  Priority=1  DataStoreName=oTilt  DataStoreElements=oTilt.oMot_.oParam_.fPwmFreqKhz_  IndexOptions=Index vector (dialog)  Indices=1  OutputSizes=1
  Data Store Write1 : DataStoreWrite  Priority=1  DataStoreName=oTilt  DataStoreElements=oTilt.oMot_.oParam_.fPwmPeriodTicksMainloopFloat_  IndexOptions=Index vector (dialog)  Indices=1  OutputSizes=1
  Data Store Write2 : DataStoreWrite  Priority=1  DataStoreName=oTilt  DataStoreElements=oTilt.oIsr_.oParam_.fPwmPeriodTicksFloat_  IndexOptions=Index vector (dialog)  Indices=1  OutputSizes=1
  Data Store Write3 : DataStoreWrite  Priority=1  DataStoreName=oTilt  DataStoreElements=oTilt.oIsr_.oParam_.fControlLoopDt_  IndexOptions=Index vector (dialog)  Indices=1  OutputSizes=1
  Data Store Write4 : DataStoreWrite  Priority=1  DataStoreName=oTilt  DataStoreElements=oTilt.oMot_.oParam_.fIntControlLoopDt_  IndexOptions=Index vector (dialog)  Indices=1  OutputSizes=1
  Data Store Write5 : DataStoreWrite  Priority=15  DataStoreName=oTilt  DataStoreElements=oTilt.oMot_.oState_.fMotorAccelerationStage1Bandwidth_  IndexOptions=Index vector (dialog)  Indices=1  OutputSizes=1
  Data Store Write6 : DataStoreWrite  Priority=15  DataStoreName=oTilt  DataStoreElements=oTilt.oMot_.oState_.fFilterBandwidthForSpeedControlIqRef_  IndexOptions=Index vector (dialog)  Indices=1  OutputSizes=1
  Data Type Conversion : DataTypeConversion  OutDataTypeStr=double
  Divide : Product  Priority=1  Inputs=/*
  Divide1 : Product  Priority=1  Inputs=/*
  Divide2 : Product  Priority=1  Inputs=*/
  Saturation : Saturate  Priority=1  UpperLimit=PWM_FREQ_KHZ__PROP  LowerLimit=1.5
  softwareIirFilterInitialize() : Subsystem  Priority=15  TreatAsAtomicUnit=on
  softwareIirFilterInitialize()1 : Subsystem  Priority=15  TreatAsAtomicUnit=on
  updateObserver()_tilt : Subsystem  Priority=5  TreatAsAtomicUnit=on
  updateServoObserver()_tilt : Subsystem  Priority=10  TreatAsAtomicUnit=on
  wires:
  Data Type Conversion/1 -> updateServoObserver()_tilt/1(oIsr_.oParam_.fControlLoopDt_)
  Data Store Read2/1 -> updateServoObserver()_tilt/2(fOmegaEDifferentiatorBandwidthHz_)
  Data Store Read1/1 -> updateObserver()_tilt/2(fObserverLoopFilterBandwidthHz_)
  Constant1/1 -> Divide1/2
  Constant2/1 -> Divide2/1
  softwareIirFilterInitialize()/1(fActualFrequencyHz) -> Data Store Write5/1
  Divide1/1 -> Data Store Write3/1, Data Store Write4/1, updateObserver()_tilt/1(oIsr_.oParam_.fControlLoopDt_), Data Type Conversion/1, Divide2/2
  Constant/1 -> Divide/2
  Divide/1 -> Data Store Write2/1, Data Store Write1/1
  softwareIirFilterInitialize()1/1(fActualFrequencyHz) -> Data Store Write6/1
  Saturation/1 -> Data Store Write/1, Divide1/1, Divide/1
  fMotorAccelerationStage1Bandwidth_/1 -> softwareIirFilterInitialize()/1(fFreq3db)
  Divide2/1 -> softwareIirFilterInitialize()/2(fFreqSample), softwareIirFilterInitialize()1/2(fFreqSample)
  fPwmFreqKhz_/1 -> Saturation/1
  fFilterBandwidthForSpeedControlIqRef_/1 -> softwareIirFilterInitialize()1/1(fFreq3db)

== system Target_Control_System/Target_Control_System/Simulation Controls/Simulation Data Store Initialization/setupPwm(&oTilt)/setPwmFrequencyApplication()_tilt/updateObserver()_tilt ==
  oIsr_.oParam_.fControlLoopDt_ : Inport
  fObserverLoopFilterBandwidthHz_ : Inport  Port=2
  Constant : Constant  Value=15*2*pi  OutDataTypeStr=single
  Constant1 : Constant  Value=8*2*pi  OutDataTypeStr=single
  Constant2 : Constant  Value=2*pi  OutDataTypeStr=single
  Constant3 : Constant  Value=500  OutDataTypeStr=single
  Constant4 : Constant  Value=20  OutDataTypeStr=single
  Constant5 : Constant  Value=100*2*pi  OutDataTypeStr=single
  Constant6 : Constant  Value=4*2*pi  OutDataTypeStr=single
  Constant7 : Constant  Value=0.0625  OutDataTypeStr=single
  Data Store Write : DataStoreWrite  DataStoreName=oTilt  DataStoreElements=oTilt.oIsr_.oParam_.fALpf4hpfDcBlocking_  IndexOptions=Index vector (dialog)  Indices=1  OutputSizes=1
  Data Store Write1 : DataStoreWrite  DataStoreName=oTilt  DataStoreElements=oTilt.oIsr_.oParam_.fAFluxMagnitude_  IndexOptions=Index vector (dialog)  Indices=1  OutputSizes=1
  Data Store Write2 : DataStoreWrite  DataStoreName=oTilt  DataStoreElements=oTilt.oIsr_.oParam_.fALoopfilter2_  IndexOptions=Index vector (dialog)  Indices=1  OutputSizes=1
  Data Store Write3 : DataStoreWrite  DataStoreName=oTilt  DataStoreElements=oTilt.oMot_.oParam_.fObserverLoopFilterBandwidthHz_  IndexOptions=Index vector (dialog)  Indices=1  OutputSizes=1
  Data Store Write4 : DataStoreWrite  DataStoreName=oTilt  DataStoreElements=oTilt.oIsr_.oParam_.fAOmegaFilter2_  IndexOptions=Index vector (dialog)  Indices=1  OutputSizes=1
  Data Store Write5 : DataStoreWrite  DataStoreName=oTilt  DataStoreElements=oTilt.oMot_.oParam_.fAOmegaXfilter2_  IndexOptions=Index vector (dialog)  Indices=1  OutputSizes=1
  Data Store Write6 : DataStoreWrite  DataStoreName=oTilt  DataStoreElements=oTilt.oIsr_.oParam_.oPiDataPll2_.oParameter_.fKp_  IndexOptions=Index vector (dialog)  Indices=1  OutputSizes=1
  Divide{,1,3..4} (4 alike) : Product  Inputs=**
  Divide2 : Product  Inputs=***
  Divide5 : Product  Inputs=*/
  GreaterThan : RelationalOperator  Operator=<  OutDataTypeStr=boolean  RndMeth=Simplest
  Saturation{,1..4} (5 alike) : Saturate  UpperLimit=1.0  LowerLimit=1e-6
  Switch : Switch  Criteria=u2 > Threshold
  wires:
  Divide5/1 -> Data Store Write6/1
  Constant7/1 -> Divide5/1
  Saturation4/1 -> Data Store Write5/1
  oIsr_.oParam_.fControlLoopDt_/1 -> Divide/1, Divide1/1, Divide3/1, Divide2/2, Divide5/2, Divide4/1
  Divide4/1 -> Saturation4/1
  Constant6/1 -> Divide4/2
  Saturation3/1 -> Data Store Write4/1
  Divide3/1 -> Saturation3/1
  Constant5/1 -> Divide3/2
  Switch/1 -> Data Store Write3/1, Divide2/1
  Constant3/1 -> Switch/1
  GreaterThan/1 -> Switch/2
  Constant4/1 -> GreaterThan/2
  fObserverLoopFilterBandwidthHz_/1 -> Switch/3, GreaterThan/1
  Divide2/1 -> Saturation2/1
  Saturation2/1 -> Data Store Write2/1
  Constant2/1 -> Divide2/3
  Divide1/1 -> Saturation1/1
  Saturation1/1 -> Data Store Write1/1
  Constant1/1 -> Divide1/2
  Saturation/1 -> Data Store Write/1
  Divide/1 -> Saturation/1
  Constant/1 -> Divide/2

== system Target_Control_System/Target_Control_System/Simulation Controls/Simulation Data Store Initialization/setupPwm()/setPwmFrequencyApplication()_pitch/setPwmFrequency()_pitch ==
  fPwmFreqKhz_ : Inport
  fMotorAccelerationStage1Bandwidth_ : Inport  Port=2
  fFilterBandwidthForSpeedControlIqRef_ : Inport  Port=3
  Constant : Constant  Priority=1  Value=50000  OutDataTypeStr=single  SampleTime=-1
  Constant1 : Constant  Priority=1  Value=0.0005  OutDataTypeStr=single  SampleTime=-1
  Constant2 : Constant  Priority=1  OutDataTypeStr=single  SampleTime=-1
  Data Store Read1 : DataStoreRead  Priority=1  DataStoreName=oPitch  DataStoreElements=oPitch.oMot_.oParam_.fObserverLoopFilterBandwidthHz_  IndexOptions=Index vector (dialog)  Indices=1  OutputSizes=1
  Data Store Read2 : DataStoreRead  Priority=1  DataStoreName=oPitch  DataStoreElements=oPitch.oMot_.oState_.oPosSensor_.fOmegaEDifferentiatorBandwidthHz_  IndexOptions=Index vector (dialog)  Indices=1  OutputSizes=1
  Data Store Write : DataStoreWrite  Priority=1  DataStoreName=oPitch  DataStoreElements=oPitch.oMot_.oParam_.fPwmFreqKhz_  IndexOptions=Index vector (dialog)  Indices=1  OutputSizes=1
  Data Store Write1 : DataStoreWrite  Priority=1  DataStoreName=oPitch  DataStoreElements=oPitch.oMot_.oParam_.fPwmPeriodTicksMainloopFloat_  IndexOptions=Index vector (dialog)  Indices=1  OutputSizes=1
  Data Store Write2 : DataStoreWrite  Priority=1  DataStoreName=oPitch  DataStoreElements=oPitch.oIsr_.oParam_.fPwmPeriodTicksFloat_  IndexOptions=Index vector (dialog)  Indices=1  OutputSizes=1
  Data Store Write3 : DataStoreWrite  Priority=1  DataStoreName=oPitch  DataStoreElements=oPitch.oIsr_.oParam_.fControlLoopDt_  IndexOptions=Index vector (dialog)  Indices=1  OutputSizes=1
  Data Store Write4 : DataStoreWrite  Priority=1  DataStoreName=oPitch  DataStoreElements=oPitch.oMot_.oParam_.fIntControlLoopDt_  IndexOptions=Index vector (dialog)  Indices=1  OutputSizes=1
  Data Store Write5 : DataStoreWrite  Priority=15  DataStoreName=oPitch  DataStoreElements=oPitch.oMot_.oState_.fMotorAccelerationStage1Bandwidth_  IndexOptions=Index vector (dialog)  Indices=1  OutputSizes=1
  Data Store Write6 : DataStoreWrite  Priority=15  DataStoreName=oPitch  DataStoreElements=oPitch.oMot_.oState_.fFilterBandwidthForSpeedControlIqRef_  IndexOptions=Index vector (dialog)  Indices=1  OutputSizes=1
  Data Type Conversion : DataTypeConversion  OutDataTypeStr=double
  Divide : Product  Priority=1  Inputs=/*
  Divide1 : Product  Priority=1  Inputs=/*
  Divide2 : Product  Priority=1  Inputs=*/
  Saturation : Saturate  Priority=1  UpperLimit=PWM_FREQ_KHZ__PROP  LowerLimit=1.5
  softwareIirFilterInitialize() : Subsystem  Priority=15  TreatAsAtomicUnit=on
  softwareIirFilterInitialize()1 : Subsystem  Priority=15  TreatAsAtomicUnit=on
  updateObserver()_pitch : Subsystem  Priority=5  TreatAsAtomicUnit=on
  updateServoObserver()_pitch : Subsystem  Priority=10  TreatAsAtomicUnit=on
  wires:
  Data Type Conversion/1 -> updateServoObserver()_pitch/1(oIsr_.oParam_.fControlLoopDt_)
  Data Store Read2/1 -> updateServoObserver()_pitch/2(fOmegaEDifferentiatorBandwidthHz_)
  Data Store Read1/1 -> updateObserver()_pitch/2(fObserverLoopFilterBandwidthHz_)
  Constant1/1 -> Divide1/2
  Constant2/1 -> Divide2/1
  softwareIirFilterInitialize()/1(fActualFrequencyHz) -> Data Store Write5/1
  Divide1/1 -> Data Store Write3/1, Data Store Write4/1, updateObserver()_pitch/1(oIsr_.oParam_.fControlLoopDt_), Data Type Conversion/1, Divide2/2
  Constant/1 -> Divide/2
  Divide/1 -> Data Store Write2/1, Data Store Write1/1
  softwareIirFilterInitialize()1/1(fActualFrequencyHz) -> Data Store Write6/1
  Saturation/1 -> Data Store Write/1, Divide1/1, Divide/1
  fMotorAccelerationStage1Bandwidth_/1 -> softwareIirFilterInitialize()/1(fFreq3db)
  Divide2/1 -> softwareIirFilterInitialize()/2(fFreqSample), softwareIirFilterInitialize()1/2(fFreqSample)
  fPwmFreqKhz_/1 -> Saturation/1
  fFilterBandwidthForSpeedControlIqRef_/1 -> softwareIirFilterInitialize()1/1(fFreq3db)
